simulink model "Model_Platform"  (R2018a)
settings: Solver=ode1  StartTime=0.0  StopTime=inf  FixedStep=0.001  RelTol=1e-3  EnableMultiTasking=on
PreLoadFcn:
  | ;HLABlocksetInit;;HLABlocksetInit;;HLABlocksetInit;
PostLoadFcn:
  | ;set_param(gcs,'PostCodeGenCommand', 'rtw_defines(buildInfo)');;set_param(gcs,'PostCodeGenCommand', 'rtw_defines(buildInfo)');;set_param(gcs,'PostCodeGenCommand', 'rtw_defines(buildInfo)');
undefined symbols (not defined in the file or in its folder): eng_speed, Heading_init, inertiaLateral, Joystick, Newton, omega_engine, omega_max, omega_wheel, Para, radiusWheel, Raphson, Standard_Devices, torque, Torque_lost, Torque_lost_wheel, X_init, Y_init, Z_init
libraries: simulink x26, dspnetwork x4, rtwinlib x2, PC_Simulator_Lib x2, vrlib x1
(part 2 of 4)

== system Model_Platform/Vehicle model/Vehicle dynamics/velocity ==
  longitudenal_velocity_Vx : Inport
  Lateral_velocity_Vy : Inport  Port=2
  rate_of_change_Yaw_Angle : Inport  Port=3
  angel_of_rotation_of_front_left_wheel : Inport  Port=4
  angel_of_rotation_of_front_Right_wheel : Inport  Port=5
  Mux2 : Mux
  Mux3 : Mux
  R : Subsystem
  to_tire : Subsystem
  velocity_at_Front_Left : Subsystem
  velocity_at_Front_Right : Subsystem
  velocity_at_Rear_Left : Subsystem
  velocity_at_Rear_Right : Subsystem
  velocity_conditioning : Subsystem
  velocity_at_wheels_in_X_mux(4) : Outport
  velocity_at_wheels_in_Y_mux(4) : Outport  Port=2
  R_CG : Outport  Port=3
  wires:
  velocity_conditioning/3(R_CGout) -> R_CG/1
  to_tire/2(velocity_at_wheels_in_Y_mux(4)final) -> velocity_at_wheels_in_Y_mux(4)/1
  to_tire/1(velocity_at_wheels_in_X_mux(4)final) -> velocity_at_wheels_in_X_mux(4)/1
  angel_of_rotation_of_front_Right_wheel/1 -> to_tire/2(angel_of_rotation_of_front_Right_wheel)
  angel_of_rotation_of_front_left_wheel/1 -> to_tire/1(angel_of_rotation_of_front_left_wheel)
  velocity_conditioning/1(velocity_at_wheels_in_X_mux(4)out) -> to_tire/3(velocity_at_wheels_in_X_mux(4))
  velocity_conditioning/2(velocity_at_wheels_in_Y_mux(4)out) -> to_tire/4(velocity_at_wheels_in_Y_mux(4))
  Mux2/1 -> velocity_conditioning/1(velocity_at_wheels_in_X_mux(4)in)
  Mux3/1 -> velocity_conditioning/2(velocity_at_wheels_in_Y_mux(4)in)
  R/1(R_CG) -> velocity_conditioning/3(R_CGin)
  Lateral_velocity_Vy/1 -> velocity_conditioning/5(VyCG), velocity_at_Front_Right/3(Lateral_velocity_Vy), R/3(Lateral_velocity_Vy), velocity_at_Rear_Right/3(Lateral_velocity_Vy), velocity_at_Rear_Left/3(Lateral_velocity_Vy), velocity_at_Front_Left/3(Lateral_velocity_Vy)
  velocity_at_Rear_Left/3(slip_angel_at_Rear_left) -> R/1(slip_angel_at_Rear_left)
  velocity_at_Rear_Right/2(velocity_at_Rear_Right_in_Y) -> Mux3/4
  velocity_at_Rear_Left/2(velocity_at_Rear_left_in_Y) -> Mux3/3
  velocity_at_Front_Left/2(velocity_at_Front_left_in_Y) -> Mux3/1
  velocity_at_Front_Right/2(velocity_at_Front_Right_in_Y) -> Mux3/2
  velocity_at_Rear_Right/1(velocity_at_Rear_Right_in_X) -> Mux2/4
  velocity_at_Rear_Left/1(velocity_at_Rear_left_in_X) -> Mux2/3
  velocity_at_Front_Right/1(velocity_at_Front_Right_in_X) -> Mux2/2
  velocity_at_Front_Left/1(velocity_at_Front_left_in_X) -> Mux2/1
  longitudenal_velocity_Vx/1 -> velocity_conditioning/4(VxCG), velocity_at_Front_Right/2(longitudenal_velocity_Vx), R/2(longitudenal_velocity_Vx), velocity_at_Rear_Right/2(longitudenal_velocity_Vx), velocity_at_Rear_Left/2(longitudenal_velocity_Vx), velocity_at_Front_Left/2(longitudenal_velocity_Vx)
  rate_of_change_Yaw_Angle/1 -> velocity_at_Front_Right/1(rate_of_change_Yaw_Angle), velocity_at_Rear_Right/1(rate_of_change_Yaw_Angle), velocity_at_Rear_Left/1(rate_of_change_Yaw_Angle), velocity_at_Front_Left/1(rate_of_change_Yaw_Angle)

== system Model_Platform/Vehicle model/Vehicle dynamics/xy_Global ==
  note: yaw_vehicle
  Vx_CG : Inport
  Vy_CG : Inport  Port=2
  rate_of_change_Yaw_Angle : Inport  Port=3
  Add8 : Sum  Inputs=+-
  Add9 : Sum
  Integrator1 : Integrator  InitialCondition=Heading_init
  Integrator8 : Integrator  InitialCondition=X_init
  Integrator9 : Integrator  InitialCondition=Y_init
  Product{16..19} (4 alike) : Product  RndMeth=Zero
  Trigonometric Function : Trigonometry  Operator=cos
  Trigonometric Function1 : Trigonometry
  Vx_global : Outport
  Vy_global : Outport  Port=2
  x_CG : Outport  Port=3
  y_CG : Outport  Port=4
  Actual_YAW : Outport  Port=5
  wires:
  Add9/1 -> Vy_global/1, Integrator9/1
  Integrator8/1 -> x_CG/1
  rate_of_change_Yaw_Angle/1 -> Integrator1/1
  Integrator1/1 -> Trigonometric Function1/1, Trigonometric Function/1, Actual_YAW/1
  Vx_CG/1 -> Product16/1, Product18/1
  Vy_CG/1 -> Product17/1, Product19/2
  Add8/1 -> Vx_global/1, Integrator8/1
  Product16/1 -> Add8/1
  Product17/1 -> Add8/2
  Product19/1 -> Add9/2
  Product18/1 -> Add9/1
  Integrator9/1 -> y_CG/1
  Trigonometric Function/1 -> Product19/1, Product16/2
  Trigonometric Function1/1 -> Product17/2, Product18/2

== system Model_Platform/Vehicle model/Drive_Train/4_Wheels_drive_train_and_Brake/Brake ==
  Feedback : Inport
  Add : Sum
  Bus Selector1 : BusSelector  OutputSignals=Vehicle_Dynamics.Vx_COG[m|s]
  Bus Selector6 : BusSelector  OutputSignals=Driver_Interface.Brake_Pedal_norm
  Compare To Constant : simulink/Logic and Bit Operations/Compare To Constant  relop=>=  const=0.7  OutDataTypeStr=uint8
  Compare To Constant1 : simulink/Logic and Bit Operations/Compare To Constant  relop=<=  const=-1  OutDataTypeStr=uint8
  Compare To Constant2 : simulink/Logic and Bit Operations/Compare To Constant  relop=<  const=0  OutDataTypeStr=uint8
  Constant1 : Constant  Value=0.35
  Constant2 : Constant
  Data Type Conversion : DataTypeConversion
  Data Type Conversion1 : DataTypeConversion
  Ground : Ground
  Ground1 : Ground
  Logical Operator : Logic  Operator=OR  AllPortsSameDT=off  OutDataTypeStr=boolean
  Product : Product  Inputs=5  RndMeth=Zero
  Product1 : Product  RndMeth=Zero
  Saturation : Saturate  UpperLimit=1  LowerLimit=0
  Sign : Signum
  Subsystem : Subsystem
  Subsystem1 : Subsystem
  Switch : Switch  Criteria=u2 > Threshold
  Terminator : Terminator
  Torque_max : Constant  Value=Para.DT.Torque_max_Brake.v
  Torque_Brake_Nm : Outport
  wires:
  Subsystem1/1(Out1) -> Add/2
  Add/1 -> Torque_Brake_Nm/1
  Product/1 -> Add/1
  Compare To Constant1/1 -> Logical Operator/2
  Data Type Conversion/1 -> Product/3
  Constant2/1 -> Switch/3, Product/5
  Switch/1 -> Product/4
  Product1/1 -> Product/1
  Constant1/1 -> Switch/1
  Data Type Conversion1/1 -> Switch/2
  Compare To Constant2/1 -> Data Type Conversion1/1
  Saturation/1 -> Subsystem1/2(Brake_Pedal[norm]), Product1/2
  Torque_max/1 -> Product1/1
  Feedback/1 -> Bus Selector6/1, Bus Selector1/1
  Bus Selector1/1 -> Sign/1, Compare To Constant2/1, Subsystem1/1(v_X_CoG[m|s]), Compare To Constant1/1, Compare To Constant/1  "<Vx_COG[m|s]>"
  Sign/1 -> Product/2
  Bus Selector6/1 -> Saturation/1  "<Brake_Pedal_norm>"
  Compare To Constant/1 -> Logical Operator/1
  Logical Operator/1 -> Data Type Conversion/1
  Subsystem/1(Torque_Brake_act_Nm) -> Terminator/1
  Ground/1 -> Subsystem/1(Torque_Brake_Nm)
  Ground1/1 -> Subsystem/2(Omega_rad/s)

== system Model_Platform/Vehicle model/Drive_Train/4_Wheels_drive_train_and_Brake/FL ==
  F_z : Inport
  Vx : Inport  Port=2
  Vy : Inport  Port=3
  Coeffecient_of_friction : Inport  Port=4
  Torque_Drive_Nm : Inport  Port=5
  Torque_Brake_Nm : Inport  Port=6
  Alpha_Kappa_Selector2 : Subsystem
  Fx_calculator : MATLAB Function  TreatAsAtomicUnit=on
  Fy_calculator : MATLAB Function  TreatAsAtomicUnit=on
  Radius_of_tire : Constant  Value=radiusWheel
  Wheel dynamics : Subsystem
  Fx : Outport
  Fy : Outport  Port=2
  Omega : Outport  Port=3
  omegaDot_radPs2 : Outport  Port=4
  wires:
  Alpha_Kappa_Selector2/2(alpha) -> Fx_calculator/2(alpha), Fy_calculator/2(alpha)
  Alpha_Kappa_Selector2/1(kappa) -> Fy_calculator/1(lambda), Fx_calculator/1(lambda)
  Torque_Brake_Nm/1 -> Wheel dynamics/3(Torque_Brake_Nm)
  Torque_Drive_Nm/1 -> Wheel dynamics/2(Torque_Drive_Nm)
  Wheel dynamics/2(omegaDot_radPs2) -> omegaDot_radPs2/1
  Fx_calculator/1(Fx) -> Alpha_Kappa_Selector2/5(Fx), Fx/1, Wheel dynamics/1(F_x)  "F_long"
  Coeffecient_of_friction/1 -> Fx_calculator/4(mue), Fy_calculator/5(mue)
  Fy_calculator/1(Fy) -> Fy/1
  F_z/1 -> Fx_calculator/3(Fz), Fy_calculator/4(Fz)
  Vy/1 -> Alpha_Kappa_Selector2/2(Vy)
  Radius_of_tire/1 -> Alpha_Kappa_Selector2/4(Rdyn)
  Vx/1 -> Alpha_Kappa_Selector2/1(Vx), Fy_calculator/3(V_x)
  Wheel dynamics/1(omega_radPs) -> Alpha_Kappa_Selector2/3(omega), Omega/1

== system Model_Platform/Vehicle model/Drive_Train/4_Wheels_drive_train_and_Brake/FR ==
  F_z : Inport
  Vx : Inport  Port=2
  Vy : Inport  Port=3
  Coeffecient_of_friction : Inport  Port=4
  Torque_Drive_Nm : Inport  Port=5
  Torque_Brake_Nm : Inport  Port=6
  Alpha_Kappa_Selector2 : Subsystem
  Fx_calculator : MATLAB Function  TreatAsAtomicUnit=on
  Fy_calculator : MATLAB Function  TreatAsAtomicUnit=on
  Radius_of_tire : Constant  Value=radiusWheel
  Wheel dynamics : Subsystem
  Fx : Outport
  Fy : Outport  Port=2
  Omega : Outport  Port=3
  omegaDot_radPs2 : Outport  Port=4
  wires:
  Torque_Brake_Nm/1 -> Wheel dynamics/3(Torque_Brake_Nm)
  Torque_Drive_Nm/1 -> Wheel dynamics/2(Torque_Drive_Nm)
  Wheel dynamics/2(omegaDot_radPs2) -> omegaDot_radPs2/1
  Fx_calculator/1(Fx) -> Fx/1, Wheel dynamics/1(F_x), Alpha_Kappa_Selector2/5(Fx)  "F_long"
  Coeffecient_of_friction/1 -> Fx_calculator/4(mue), Fy_calculator/5(mue)
  Fy_calculator/1(Fy) -> Fy/1
  Alpha_Kappa_Selector2/1(kappa) -> Fx_calculator/1(lambda), Fy_calculator/1(lambda)
  Alpha_Kappa_Selector2/2(alpha) -> Fy_calculator/2(alpha), Fx_calculator/2(alpha)
  F_z/1 -> Fx_calculator/3(Fz), Fy_calculator/4(Fz)
  Vy/1 -> Alpha_Kappa_Selector2/2(Vy)
  Radius_of_tire/1 -> Alpha_Kappa_Selector2/4(Rdyn)
  Vx/1 -> Fy_calculator/3(V_x), Alpha_Kappa_Selector2/1(Vx)
  Wheel dynamics/1(omega_radPs) -> Omega/1, Alpha_Kappa_Selector2/3(omega)

== system Model_Platform/Vehicle model/Drive_Train/4_Wheels_drive_train_and_Brake/RL ==
  F_z : Inport
  Vx : Inport  Port=2
  Vy : Inport  Port=3
  Coeffecient_of_friction : Inport  Port=4
  Torque_Drive_Nm : Inport  Port=5
  Torque_Brake_Nm : Inport  Port=6
  Alpha_Kappa_Selector2 : Subsystem
  Fx_calculator : MATLAB Function  TreatAsAtomicUnit=on
  Fy_calculator : MATLAB Function  TreatAsAtomicUnit=on
  Radius_of_tire : Constant  Value=radiusWheel
  Wheel dynamics : Subsystem
  Fx : Outport
  Fy : Outport  Port=2
  Omega : Outport  Port=3
  omegaDot_radPs2 : Outport  Port=4
  wires:
  Torque_Brake_Nm/1 -> Wheel dynamics/3(Torque_Brake_Nm)
  Torque_Drive_Nm/1 -> Wheel dynamics/2(Torque_Drive_Nm)
  Wheel dynamics/2(omegaDot_radPs2) -> omegaDot_radPs2/1
  Fx_calculator/1(Fx) -> Alpha_Kappa_Selector2/5(Fx), Fx/1, Wheel dynamics/1(F_x)  "F_long"
  Coeffecient_of_friction/1 -> Fx_calculator/4(mue), Fy_calculator/5(mue)
  Fy_calculator/1(Fy) -> Fy/1
  Alpha_Kappa_Selector2/1(kappa) -> Fx_calculator/1(lambda), Fy_calculator/1(lambda)
  Alpha_Kappa_Selector2/2(alpha) -> Fy_calculator/2(alpha), Fx_calculator/2(alpha)
  F_z/1 -> Fx_calculator/3(Fz), Fy_calculator/4(Fz)
  Vy/1 -> Alpha_Kappa_Selector2/2(Vy)
  Radius_of_tire/1 -> Alpha_Kappa_Selector2/4(Rdyn)
  Vx/1 -> Fy_calculator/3(V_x), Alpha_Kappa_Selector2/1(Vx)
  Wheel dynamics/1(omega_radPs) -> Alpha_Kappa_Selector2/3(omega), Omega/1

== system Model_Platform/Vehicle model/Drive_Train/4_Wheels_drive_train_and_Brake/RR ==
  F_z : Inport
  Vx : Inport  Port=2
  Vy : Inport  Port=3
  Coeffecient_of_friction : Inport  Port=4
  Torque_Drive_Nm : Inport  Port=5
  Torque_Brake_Nm : Inport  Port=6
  Alpha_Kappa_Selector2 : Subsystem
  Fx_calculator : MATLAB Function  TreatAsAtomicUnit=on
  Fy_calculator : MATLAB Function  TreatAsAtomicUnit=on
  Radius_of_tire : Constant  Value=radiusWheel
  Wheel dynamics : Subsystem
  Fx : Outport
  Fy : Outport  Port=2
  Omega : Outport  Port=3
  omegaDot_radPs2 : Outport  Port=4
  wires:
  Torque_Brake_Nm/1 -> Wheel dynamics/3(Torque_Brake_Nm)
  Torque_Drive_Nm/1 -> Wheel dynamics/2(Torque_Drive_Nm)
  Wheel dynamics/2(omegaDot_radPs2) -> omegaDot_radPs2/1
  Fx_calculator/1(Fx) -> Alpha_Kappa_Selector2/5(Fx), Fx/1, Wheel dynamics/1(F_x)  "F_long"
  Coeffecient_of_friction/1 -> Fx_calculator/4(mue), Fy_calculator/5(mue)
  Fy_calculator/1(Fy) -> Fy/1
  Alpha_Kappa_Selector2/1(kappa) -> Fx_calculator/1(lambda), Fy_calculator/1(lambda)
  Alpha_Kappa_Selector2/2(alpha) -> Fy_calculator/2(alpha), Fx_calculator/2(alpha)
  F_z/1 -> Fx_calculator/3(Fz), Fy_calculator/4(Fz)
  Vy/1 -> Alpha_Kappa_Selector2/2(Vy)
  Radius_of_tire/1 -> Alpha_Kappa_Selector2/4(Rdyn)
  Vx/1 -> Alpha_Kappa_Selector2/1(Vx), Fy_calculator/3(V_x)
  Wheel dynamics/1(omega_radPs) -> Alpha_Kappa_Selector2/3(omega), Omega/1

== system Model_Platform/Vehicle model/HMI_Realtime_normal_mode/HMI_Logitech1/Subsystem1 ==
  In1 : Inport
  Compare To Constant : simulink/Logic and Bit Operations/Compare To Constant  relop=>=  const=0.0001  OutDataTypeStr=boolean
  Constant : Constant
  Data Type Conversion : DataTypeConversion
  Gain : Gain
  Product : Product
  Sum : Sum  Inputs=|-+
  Out1 : Outport
  wires:
  Data Type Conversion/1 -> Product/2
  Compare To Constant/1 -> Data Type Conversion/1
  Product/1 -> Out1/1
  In1/1 -> Sum/1
  Sum/1 -> Gain/1
  Constant/1 -> Sum/2
  Gain/1 -> Product/1, Compare To Constant/1

== system Model_Platform/Vehicle model/HMI_Realtime_normal_mode/HMI_Logitech1/Subsystem2 ==
  In1 : Inport
  Compare To Constant : simulink/Logic and Bit Operations/Compare To Constant  relop=>=  const=0.0001  OutDataTypeStr=boolean
  Constant : Constant
  Data Type Conversion : DataTypeConversion
  Gain : Gain  Gain=.5
  Product : Product
  Sum : Sum  Inputs=|-+
  Out1 : Outport
  wires:
  Data Type Conversion/1 -> Product/2
  Compare To Constant/1 -> Data Type Conversion/1
  Product/1 -> Out1/1
  In1/1 -> Sum/1
  Sum/1 -> Gain/1
  Constant/1 -> Sum/2
  Gain/1 -> Product/1, Compare To Constant/1

== system Model_Platform/Vehicle model/Vehicle dynamics/Forces_transformation/Force_of_Aerodynamics ==
  note: Neglecting the air resistance effect in Y and modefing the equation
      | (V_abs*cos(slip))^2*Cd
      | insted of
      | V_abs^2*cos(slip)*Cd
      | by Berry
      | if not understud call me now
      | +20122299183
  velocity_of_car_absolut : Inport
  Slip_angle_of_velocity : Inport  Port=2
  Demux : Demux  Outputs=2
  Gain : Gain  Gain=Para.VD.Air_Risistance_Coefficient.v
  Product1 : Product  RndMeth=Zero
  Product2 : Product  RndMeth=Zero
  Product4 : Product  RndMeth=Zero
  Trigonometric Function3 : Trigonometry  Operator=cos
  Unary Minus : UnaryMinus
  Force_of_aerodynamics_in_X : Outport
  wires:
  Product2/1 -> Force_of_aerodynamics_in_X/1
  Gain/1 -> Product2/1
  Unary Minus/1 -> Product2/2
  Demux/2 -> Unary Minus/1
  Demux/1 -> Product4/1
  velocity_of_car_absolut/1 -> Demux/1
  Product1/1 -> Gain/1
  Product4/1 -> Product1/1, Product1/2
  Slip_angle_of_velocity/1 -> Trigonometric Function3/1
  Trigonometric Function3/1 -> Product4/2

== system Model_Platform/Vehicle model/Vehicle dynamics/Forces_transformation/Moment _about _Z_axis_calculation ==
  note: produce
      | the moment around Z
      | axis due to the total effect
      | of the forces acting on the
      | vehicle
  note: RR_Y
  note: RL_Y
  note: FR_Y
  note: FL_Y
  note: RR_X
  note: RL_X
  note: FR_X
  note: FL_X
  Forces_Acting_in_X_Wheels : Inport
  Forces_Acting_in_Y_Wheels : Inport  Port=2
  Add : Sum  Inputs=-++-
  Demux1 : Demux
  Demux3 : Demux
  Length_CG_Front_Wheels : Constant  Value=Para.VD.Length_Front.v
  Length_CG_Rear_Wheels : Constant  Value=Para.VD.Length_Rear.v
  Product{1..4} (4 alike) : Product  RndMeth=Zero
  Subtract{1..4} (4 alike) : Sum
  Width_of_Car/2 : Constant  Value=Para.VD.Wheel_Base_Width.v/2
  Moment _about _Z_axis : Outport
  wires:
  Add/1 -> Moment _about _Z_axis/1
  Demux3/2 -> Subtract3/1
  Demux3/3 -> Subtract4/2
  Length_CG_Rear_Wheels/1 -> Product2/2
  Length_CG_Front_Wheels/1 -> Product1/2
  Forces_Acting_in_Y_Wheels/1 -> Demux1/1
  Forces_Acting_in_X_Wheels/1 -> Demux3/1
  Width_of_Car/2/1 -> Product4/1, Product3/1
  Demux3/4 -> Subtract3/2
  Demux3/1 -> Subtract4/1
  Subtract4/1 -> Product3/2
  Subtract3/1 -> Product4/2
  Product4/1 -> Add/2
  Product3/1 -> Add/1
  Product2/1 -> Add/4
  Product1/1 -> Add/3
  Subtract1/1 -> Product2/1
  Demux1/4 -> Subtract1/2
  Demux1/3 -> Subtract1/1
  Subtract2/1 -> Product1/1
  Demux1/2 -> Subtract2/2
  Demux1/1 -> Subtract2/1

== system Model_Platform/Vehicle model/Vehicle dynamics/Forces_transformation/Moment _about _x_axis_calculation ==
  note: the total effect of forces
      | acting as a moment
      | around the X axis
  note: RR_Y
  note: RL_Y
  note: FR_Y
  note: FL_Y
  note: RR_Z
  note: RL_Z
  note: FR_Z
  note: FL_Z
  Forces_Z_Wheels : Inport
  Forces_Y_Wheels : Inport  Port=2
  Hight_Front_Left : Inport  Port=3
  Hight_Front_Right : Inport  Port=4
  Hight_Rear_Left : Inport  Port=5
  Hight_Rear_Right : Inport  Port=6
  Add1 : Sum  Inputs=+-+-
  Add2 : Sum  Inputs=++++
  Add3 : Sum
  Demux2 : Demux
  Demux3 : Demux
  Divide{9..16} (8 alike) : Product  Inputs=**
  Width_of_Car/1 : Constant  Value=Para.VD.Wheel_Base_Width.v/2
  Moment _about _X_axis1 : Outport
  wires:
  Add3/1 -> Moment _about _X_axis1/1
  Add2/1 -> Add3/2
  Add1/1 -> Add3/1
  Hight_Rear_Right/1 -> Divide16/2
  Hight_Rear_Left/1 -> Divide15/2
  Hight_Front_Right/1 -> Divide14/2
  Hight_Front_Left/1 -> Divide13/2
  Forces_Y_Wheels/1 -> Demux3/1
  Demux3/4 -> Divide16/1
  Demux3/3 -> Divide15/1
  Demux3/2 -> Divide14/1
  Demux3/1 -> Divide13/1
  Divide16/1 -> Add2/4
  Divide15/1 -> Add2/3
  Divide14/1 -> Add2/2
  Divide13/1 -> Add2/1
  Forces_Z_Wheels/1 -> Demux2/1
  Demux2/4 -> Divide12/2
  Demux2/3 -> Divide11/2
  Demux2/2 -> Divide10/2
  Demux2/1 -> Divide9/2
  Width_of_Car/1/1 -> Divide12/1, Divide11/1, Divide10/1, Divide9/1
  Divide9/1 -> Add1/1
  Divide10/1 -> Add1/2
  Divide11/1 -> Add1/3
  Divide12/1 -> Add1/4

== system Model_Platform/Vehicle model/Vehicle dynamics/Forces_transformation/Moment _about _y_axis_calculation ==
  note: the total effect of the car forces
      | represented as a moment acting on the
      | CG around Y axis
  note: RR_X
  note: RL_X
  note: FR_X
  note: FL_X
  note: RR_Z
  note: RL_Z
  note: FR_Z
  note: FL_Z
  Forces_Z_Wheels : Inport
  Forces_X_Wheels : Inport  Port=2
  Hight_Front_Left : Inport  Port=3
  Hight_Front_Right : Inport  Port=4
  Hight_Rear_Left : Inport  Port=5
  Hight_Rear_Right : Inport  Port=6
  Add1 : Sum  Inputs=--++
  Add2 : Sum  Inputs=----
  Add3 : Sum
  Demux1 : Demux
  Demux9 : Demux
  Divide{8..15} (8 alike) : Product  Inputs=**
  Length_CG_Front_Wheels : Constant  Value=Para.VD.Length_Front.v
  Length_CG_Rear_Wheels : Constant  Value=Para.VD.Length_Rear.v
  Moment _about _Y_axis2 : Outport
  wires:
  Add3/1 -> Moment _about _Y_axis2/1
  Hight_Rear_Right/1 -> Divide15/2
  Hight_Rear_Left/1 -> Divide14/2
  Hight_Front_Right/1 -> Divide13/2
  Hight_Front_Left/1 -> Divide12/2
  Forces_X_Wheels/1 -> Demux1/1
  Demux1/4 -> Divide15/1
  Demux1/3 -> Divide14/1
  Demux1/2 -> Divide13/1
  Demux1/1 -> Divide12/1
  Forces_Z_Wheels/1 -> Demux9/1
  Length_CG_Rear_Wheels/1 -> Divide11/2, Divide10/2
  Length_CG_Front_Wheels/1 -> Divide9/2, Divide8/2
  Demux9/4 -> Divide11/1
  Demux9/3 -> Divide10/1
  Demux9/2 -> Divide9/1
  Demux9/1 -> Divide8/1
  Divide15/1 -> Add2/4
  Divide14/1 -> Add2/3
  Divide13/1 -> Add2/2
  Divide12/1 -> Add2/1
  Divide11/1 -> Add1/4
  Divide10/1 -> Add1/3
  Divide9/1 -> Add1/2
  Divide8/1 -> Add1/1
  Add2/1 -> Add3/2
  Add1/1 -> Add3/1

== system Model_Platform/Vehicle model/Vehicle dynamics/Forces_transformation/Z1-->angles ==
  Z1(4) : Inport
  Constant3 : Constant  Value=-2*Para.VD.Length_Front.v
  Constant4 : Constant  Value=Para.VD.Wheel_Base_Width.v
  Demux : Demux
  Divide : Product  Inputs=*/
  Divide1 : Product  Inputs=*/
  Subtract3 : Sum  Inputs=+-
  Subtract4 : Sum  Inputs=+-
  Terminator : Terminator
  Trigonometric Function1 : Trigonometry  Operator=asin
  Trigonometric Function2 : Trigonometry  Operator=asin
  Roll_angel(z1)1 : Outport
  Pitch_angel(z1) : Outport  Port=2
  wires:
  Demux/4 -> Terminator/1
  Z1(4)/1 -> Demux/1
  Demux/1 -> Subtract3/1, Subtract4/1
  Demux/3 -> Subtract3/2
  Subtract3/1 -> Divide/1
  Constant3/1 -> Divide/2
  Divide/1 -> Trigonometric Function1/1
  Trigonometric Function1/1 -> Pitch_angel(z1)/1
  Demux/2 -> Subtract4/2
  Subtract4/1 -> Divide1/1
  Constant4/1 -> Divide1/2
  Divide1/1 -> Trigonometric Function2/1
  Trigonometric Function2/1 -> Roll_angel(z1)1/1

== system Model_Platform/Vehicle model/Vehicle dynamics/Forces_transformation/force acting in X direction ==
  note: the summation of forces
      | acting on the X direction
      | on CG
  note: Force_rear_right_in_x
  note: Force_rear_left_in_x
  note: Force_Front_Right_in_x
  note: Force_Front_Left_in_x
  Forces_Acting_In_X_Wheel : Inport
  Force_acting_in_x_from_mass : Inport  Port=2
  Force_in_x_air : Inport  Port=3
  Add : Sum  Inputs=++++++
  Demux1 : Demux
  Force_acting_on_CG_in_x : Outport
  wires:
  Add/1 -> Force_acting_on_CG_in_x/1
  Forces_Acting_In_X_Wheel/1 -> Demux1/1
  Force_in_x_air/1 -> Add/6
  Force_acting_in_x_from_mass/1 -> Add/5
  Demux1/4 -> Add/4
  Demux1/3 -> Add/3
  Demux1/2 -> Add/2
  Demux1/1 -> Add/1

== system Model_Platform/Vehicle model/Vehicle dynamics/Forces_transformation/force acting in Y direction ==
  note: the summation of forces
      | acting on the Y direction
      | on CG
  note: Force_Rear_Right_in_Y
  note: Force_Rear_Left_in_Y
  note: Force_Front_Right_in_Y
  note: Force_Front_Left_in_Y
  Forces_Acting_In_Y_Wheels : Inport
  Force_From_Mass_Y : Inport  Port=2
  Add : Sum  Inputs=+++++
  Demux2 : Demux
  Force_acting_on_CG_in_Y : Outport
  wires:
  Add/1 -> Force_acting_on_CG_in_Y/1
  Forces_Acting_In_Y_Wheels/1 -> Demux2/1
  Demux2/1 -> Add/1
  Demux2/2 -> Add/2
  Demux2/3 -> Add/3
  Demux2/4 -> Add/4
  Force_From_Mass_Y/1 -> Add/5

== system Model_Platform/Vehicle model/Vehicle dynamics/Forces_transformation/force acting in Z direction ==
  note: the summation of forces acting
      | on CG in Z direction
  Forces_Z_Wheel : Inport
  Force_Mass_Z : Inport  Port=2
  Add : Sum  Inputs=+++++
  Demux5 : Demux
  Force_acting_on_CG_in_z : Outport
  wires:
  Forces_Z_Wheel/1 -> Demux5/1
  Force_Mass_Z/1 -> Add/5
  Demux5/4 -> Add/4
  Add/1 -> Force_acting_on_CG_in_z/1
  Demux5/3 -> Add/3
  Demux5/2 -> Add/2
  Demux5/1 -> Add/1

== system Model_Platform/Vehicle model/Vehicle dynamics/Forces_transformation/inclination_effect_on_mass ==
  note: FZ_due to roll
  Roll_angle(z1) : Inport
  Pitch_angel(z1) : Inport  Port=2
  Gain : Gain  Gain=-1
  Gain1 : Gain  Gain=-1
  Product{1..4} (4 alike) : Product  RndMeth=Zero
  Trigonometric Function : Trigonometry  Operator=cos
  Trigonometric Function1 : Trigonometry  Operator=cos
  Trigonometric Function2 : Trigonometry
  Trigonometric Function3 : Trigonometry
  m * g : Constant  Value=Para.VD.Mass.v * Para.VD.gravity.v
  FZ_due_to_mass : Outport
  Fx_due_to_mass : Outport  Port=2
  Fy_due_to_mass : Outport  Port=3
  wires:
  Product1/1 -> Product4/2
  Trigonometric Function/1 -> Product4/1
  Gain1/1 -> Product1/2
  Trigonometric Function1/1 -> Gain1/1
  Product2/1 -> Fx_due_to_mass/1
  Product4/1 -> FZ_due_to_mass/1
  Gain/1 -> Fy_due_to_mass/1
  Product3/1 -> Gain/1
  Trigonometric Function3/1 -> Product3/2
  Trigonometric Function2/1 -> Product2/1
  m * g/1 -> Product2/2, Product3/1, Product1/1
  Roll_angle(z1)/1 -> Trigonometric Function3/1, Trigonometric Function1/1
  Pitch_angel(z1)/1 -> Trigonometric Function2/1, Trigonometric Function/1

== system Model_Platform/Vehicle model/Vehicle dynamics/Horizontal_Dyn/Beta_Slip_Angle_calculation ==
  note: this block is to develop the beta
      | slip angle and the absolut speed
      | with which the vehicle travels
      | considering direction of traveling
  Longitudinal_Velocity_Vx : Inport
  Longitudinal_Velocity_Vy : Inport  Port=2
  Bus Creator : BusCreator  Inputs=2
  Divide1 : Product  Inputs=/*
  Divide2 : Product  Inputs=**
  Divide3 : Product  Inputs=**
  Math Function : Math  Operator=sqrt  SaturateOnIntegerOverflow=on
  Sign : Signum
  Sum : Sum
  Trigonometric Function1 : Trigonometry  Operator=atan
  Beta_Slip_Angle : Outport
  absolute_velocity_of_car_with_direction : Outport  Port=2
  wires:
  Math Function/1 -> Bus Creator/1
  Bus Creator/1 -> absolute_velocity_of_car_with_direction/1
  Sign/1 -> Bus Creator/2
  Sum/1 -> Math Function/1
  Divide3/1 -> Sum/2
  Divide2/1 -> Sum/1
  Longitudinal_Velocity_Vy/1 -> Divide1/2, Divide3/2, Divide3/1
  Trigonometric Function1/1 -> Beta_Slip_Angle/1
  Divide1/1 -> Trigonometric Function1/1
  Longitudinal_Velocity_Vx/1 -> Divide2/1, Sign/1, Divide2/2, Divide1/1

== system Model_Platform/Vehicle model/Vehicle dynamics/Horizontal_Dyn/about_z_axis ==
  note: Yawddot
  Moment _about _Z_axis : Inport
  reset : Inport  Port=2
  1/Inertia_Vertical axis : Gain  Gain=1/Para.VD.Inertia_zz.v  OutDataTypeStr=double
  Integrator1 : Integrator  InitialCondition=Heading_init
  Integrator4 : Integrator  ExternalReset=level
  Yaw_Angular_ACC : Outport
  Yaw_angle_Velcity : Outport  Port=2
  Yaw_angle_(rad) : Outport  Port=3
  wires:
  reset/1 -> Integrator4/2
  Integrator4/1 -> Yaw_angle_Velcity/1, Integrator1/1
  Integrator1/1 -> Yaw_angle_(rad)/1
  1/Inertia_Vertical axis/1 -> Integrator4/1, Yaw_Angular_ACC/1
  Moment _about _Z_axis/1 -> 1/Inertia_Vertical axis/1

== system Model_Platform/Vehicle model/Vehicle dynamics/Horizontal_Dyn/in_x_direction ==
  note: XDDot
  Force_acting_on_CG_in_x : Inport
  Constant : Constant  Value=eps
  Integrator2 : Integrator  InitialCondition=eps
  Integrator3 : Integrator
  Mass : Gain  Gain=1/Para.VD.Mass.v
  Sum : Sum  Inputs=|++
  Longitudinal_Velocity_Vx : Outport
  Displacement_x : Outport  Port=2
  Acceleration_Ax : Outport  Port=3
  wires:
  Constant/1 -> Sum/2
  Sum/1 -> Mass/1
  Force_acting_on_CG_in_x/1 -> Sum/1
  Integrator2/1 -> Longitudinal_Velocity_Vx/1, Integrator3/1
  Mass/1 -> Acceleration_Ax/1, Integrator2/1
  Integrator3/1 -> Displacement_x/1

== system Model_Platform/Vehicle model/Vehicle dynamics/Horizontal_Dyn/in_y_direction ==
  note: YDDot
  note: Y
  note: YDot
  Force_acting_on_CG_in_y : Inport
  reset : Inport  Port=2
  Integrator2 : Integrator  ExternalReset=level
  Integrator3 : Integrator
  Mass : Gain  Gain=1/Para.VD.Mass.v
  Lateral_Velocity_Vy : Outport
  Displacement_y : Outport  Port=2
  Acceleration_Ay : Outport  Port=3
  wires:
  reset/1 -> Integrator2/2
  Integrator2/1 -> Lateral_Velocity_Vy/1, Integrator3/1
  Mass/1 -> Acceleration_Ay/1, Integrator2/1
  Force_acting_on_CG_in_y/1 -> Mass/1
  Integrator3/1 -> Displacement_y/1

== system Model_Platform/Vehicle model/Vehicle dynamics/Horizontal_Dyn/reset ==
  In1 : Inport
  Abs : Abs
  Compare To Constant : simulink/Logic and Bit Operations/Compare To Constant  relop=<=  const=0.5  OutDataTypeStr=boolean
  Out1 : Outport
  wires:
  Compare To Constant/1 -> Out1/1
  Abs/1 -> Compare To Constant/1
  In1/1 -> Abs/1

== system Model_Platform/Vehicle model/Vehicle dynamics/Horizontal_Dyn/reset1 ==
  In1 : Inport
  Abs : Abs
  Compare To Constant : simulink/Logic and Bit Operations/Compare To Constant  relop=<=  const=0.5  OutDataTypeStr=boolean
  Out1 : Outport
  wires:
  In1/1 -> Abs/1
  Abs/1 -> Compare To Constant/1
  Compare To Constant/1 -> Out1/1

== system Model_Platform/Vehicle model/Vehicle dynamics/Output_Maping/Subsystem1 ==
  Force_Suspention : Inport
  Bus Creator : BusCreator  Inputs=4
  Demux : Demux
  Fz_Wheel[N] : Outport
  wires:
  Bus Creator/1 -> Fz_Wheel[N]/1
  Demux/4 -> Bus Creator/4  "Fz_Wheel_RR[N]"
  Demux/3 -> Bus Creator/3  "Fz_Wheel_RL[N]"
  Demux/2 -> Bus Creator/2  "Fz_Wheel_FR[N]"
  Demux/1 -> Bus Creator/1  "Fz_Wheel_FL[N]"
  Force_Suspention/1 -> Demux/1

== system Model_Platform/Vehicle model/Vehicle dynamics/Output_Maping/Velocity_Wheels_Maping_Block ==
  Velocity_Wheels_X[m|s] : Inport
  Velocity_Wheels_Y[m|s] : Inport  Port=2
  Bus Creator : BusCreator  Inputs=4
  Bus Creator{3..5,7} (4 alike) : BusCreator  Inputs=2
  Demux1 : Demux
  Demux2 : Demux
  Velocity_Wheels[m|s] : Outport
  wires:
  Bus Creator/1 -> Velocity_Wheels[m|s]/1  "Velocity_Wheels[m|s]"
  Velocity_Wheels_Y[m|s]/1 -> Demux2/1
  Velocity_Wheels_X[m|s]/1 -> Demux1/1
  Demux2/4 -> Bus Creator7/2  "vy_RR"
  Demux1/4 -> Bus Creator7/1  "vx_RR[m|s]"
  Demux2/3 -> Bus Creator5/2  "vy_RL[m|s]"
  Demux1/3 -> Bus Creator5/1  "vx_RL[m|s]"
  Demux2/2 -> Bus Creator4/2  "vy_FR[m|s]"
  Demux1/2 -> Bus Creator4/1  "vx_FR[m|s]"
  Demux2/1 -> Bus Creator3/2  "vy_FL[m|s]"
  Demux1/1 -> Bus Creator3/1  "vx_FL[m|s]"
  Bus Creator7/1 -> Bus Creator/4  "v_RR[m|s]"
  Bus Creator5/1 -> Bus Creator/3  "v_RL[m|s]"
  Bus Creator4/1 -> Bus Creator/2  "v_FR[m|s]"
  Bus Creator3/1 -> Bus Creator/1  "v_FL[m|s]"

== system Model_Platform/Vehicle model/Vehicle dynamics/Vertical_Dyn./Invers_Trangnometric_conv ==
  Vertical_Displacement_Z_vehicle_corners_actual(4) : Inport
  Add3 : Sum  Inputs=++++-
  Constant3 : Constant  Value=-2*Para.VD.Length_Front.v
  Constant4 : Constant  Value=Para.VD.Wheel_Base_Width.v
  Constant5 : Constant  Value=2*Para.VD.Length_Rear.v-2*Para.VD.Length_Front.v
  Demux : Demux
  Divide : Product  Inputs=*/
  Divide1 : Product  Inputs=*/
  Gain1 : Gain  Gain=0.25
  Product3 : Product  RndMeth=Zero
  Subtract3 : Sum  Inputs=+-
  Subtract4 : Sum  Inputs=+-
  Trigonometric Function1 : Trigonometry  Operator=asin
  Trigonometric Function2 : Trigonometry  Operator=asin
  Vertical_Displacement_Z_CG_actual : Outport
  Roll_actual : Outport  Port=2
  Pitch_actual : Outport  Port=3
  wires:
  Gain1/1 -> Vertical_Displacement_Z_CG_actual/1
  Add3/1 -> Gain1/1
  Product3/1 -> Add3/5
  Constant5/1 -> Product3/2
  Demux/4 -> Add3/4
  Trigonometric Function2/1 -> Roll_actual/1
  Divide1/1 -> Trigonometric Function2/1
  Constant4/1 -> Divide1/2
  Subtract4/1 -> Divide1/1
  Demux/2 -> Add3/2, Subtract4/2
  Trigonometric Function1/1 -> Pitch_actual/1
  Divide/1 -> Product3/1, Trigonometric Function1/1
  Constant3/1 -> Divide/2
  Subtract3/1 -> Divide/1
  Demux/3 -> Add3/3, Subtract3/2
  Demux/1 -> Add3/1, Subtract4/1, Subtract3/1
  Vertical_Displacement_Z_vehicle_corners_actual(4)/1 -> Demux/1

== system Model_Platform/Vehicle model/Vehicle dynamics/Vertical_Dyn./Mass_Distribution ==
  note: Force acting on front wheels = (m*g*Rear_Length)/(Front_Length+Rear_Length)
      | Force acting on Rear wheels = m*g -  (m*g*Rear_Length)/(Front_Length+Rear_Length)
      | the mass are just dividing by the gravity
  note: RR_Z
  note: RL_Z
  note: FR_Z
  note: FL_Z
  note: Reaction_Force_Rear_Wheels
  note: Reaction_Force_Front_Wheels
  Mass*gravity_in_Z : Inport
  Abs : Abs
  Divide : Product  Inputs=*/
  Divide1 : Product  Inputs=*/
  Divide2 : Product  Inputs=*/
  Gain : Gain  Gain=0.5
  Gain1 : Gain  Gain=0.5
  Length_CG_Rear_Wheels : Constant  Value=Para.VD.Length_Rear.v
  Mass*gravity1 : Constant  Value=Para.VD.gravity.v*Para.VD.Mass.v
  Mux : Mux
  Mux1 : Mux
  Product : Product  RndMeth=Zero
  Subtract : Sum  Inputs=+-
  Terminator : Terminator
  Terminator1 : Terminator
  Wheel_Base_Length : Constant  Value=Para.VD.Wheel_Base_Length.v
  gravity : Constant  Value=Para.VD.gravity.v
  Forces_Z_Mass : Outport
  wires:
  Abs/1 -> Subtract/1, Product/1
  Mux1/1 -> Terminator/1
  Mass*gravity1/1 -> Terminator1/1
  gravity/1 -> Divide2/2, Divide1/2
  Divide1/1 -> Mux1/2, Mux1/1
  Divide2/1 -> Mux1/3, Mux1/4
  Mux/1 -> Forces_Z_Mass/1
  Gain1/1 -> Divide2/1, Mux/4, Mux/3
  Gain/1 -> Divide1/1, Mux/2, Mux/1
  Subtract/1 -> Gain1/1
  Divide/1 -> Gain/1, Subtract/2
  Wheel_Base_Length/1 -> Divide/2
  Product/1 -> Divide/1
  Length_CG_Rear_Wheels/1 -> Product/2
  Mass*gravity_in_Z/1 -> Abs/1

== system Model_Platform/Vehicle model/Vehicle dynamics/Vertical_Dyn./Trangnometric_conv ==
  note: RR
  note: RL
  note: FR
  note: FL
  note: 0.5*Lt*sin(Roll)
  note: Lr*sin(Pitch)
  note: Lf*sin(pitch)
  Vertical_Displacement_Z_CG : Inport
  Pitch : Inport  Port=2
  Roll : Inport  Port=3
  Add : Sum
  Add1 : Sum
  Add2 : Sum
  Constant : Constant  Value=Para.VD.Wheel_Base_Width.v
  Constant1 : Constant  Value=Para.VD.Length_Rear.v
  Constant2 : Constant  Value=Para.VD.Length_Front.v
  Gain : Gain  Gain=0.5
  Mux : Mux
  Product : Product  RndMeth=Zero
  Product1 : Product  RndMeth=Zero
  Product2 : Product  RndMeth=Zero
  Subtract : Sum  Inputs=+-
  Subtract1 : Sum  Inputs=+-
  Subtract2 : Sum  Inputs=+-
  Trigonometric Function : Trigonometry
  Trigonometric Function1 : Trigonometry
  Vertical_Displacement_Z_vehicle_corners(4) : Outport
  wires:
  Subtract2/1 -> Mux/4
  Add2/1 -> Mux/3
  Add1/1 -> Subtract2/1, Add2/2
  Subtract1/1 -> Mux/2
  Add/1 -> Mux/1
  Subtract/1 -> Subtract1/1, Add/2
  Vertical_Displacement_Z_CG/1 -> Add1/1, Subtract/1
  Product/1 -> Subtract2/2, Add2/1, Subtract1/2, Add/1
  Product2/1 -> Add1/2
  Product1/1 -> Subtract/2
  Constant2/1 -> Product1/1
  Constant1/1 -> Product2/1
  Trigonometric Function/1 -> Product1/2, Product2/2
  Trigonometric Function1/1 -> Product/1
  Gain/1 -> Product/2
  Roll/1 -> Trigonometric Function1/1
  Pitch/1 -> Trigonometric Function/1
  Constant/1 -> Gain/1
  Mux/1 -> Vertical_Displacement_Z_vehicle_corners(4)/1

== system Model_Platform/Vehicle model/Vehicle dynamics/Vertical_Dyn./Vertical_movement ==
  Vertical_Force_CG : Inport
  Moment_Y-axis_CG : Inport  Port=2
  Moment_X-axis_CG : Inport  Port=3
  1/Ixx : Gain  Gain=1/Para.VD.Inertia_xx.v
  1/Iyy : Gain  Gain=1/Para.VD.Inertia_yy.v
  1/mass : Gain  Gain=1/Para.VD.Mass.v
  Integrator{1..6} (6 alike) : Integrator
  Vertical_Displacement_Z_CG : Outport
  Pitch : Outport  Port=2
  Roll : Outport  Port=3
  Vertical_Velocity_Z_CG[m|s] : Outport  Port=4
  wires:
  Integrator1/1 -> Vertical_Displacement_Z_CG/1
  1/Ixx/1 -> Integrator5/1
  1/Iyy/1 -> Integrator3/1
  Integrator5/1 -> Integrator4/1
  Integrator3/1 -> Integrator2/1
  Integrator2/1 -> Pitch/1
  Integrator4/1 -> Roll/1
  Integrator6/1 -> Vertical_Velocity_Z_CG[m|s]/1, Integrator1/1
  1/mass/1 -> Integrator6/1
  Moment_X-axis_CG/1 -> 1/Ixx/1
  Moment_Y-axis_CG/1 -> 1/Iyy/1
  Vertical_Force_CG/1 -> 1/mass/1

== system Model_Platform/Vehicle model/Vehicle dynamics/Vertical_Dyn./suspention_System ==
  Vertical_Displacement_Z2_vehicle_corners(4) : Inport
  Vertical_Displacement_Z0(4) : Inport  Port=2
  intial_force_from_mass_Wheels(4) : Inport  Port=3
  Demux : Demux
  Demux1 : Demux
  Demux3 : Demux
  Mux{,1..3} (4 alike) : Mux
  Rear_Right_Suspention : Subsystem
  Rear_left_Suspention : Subsystem
  front_left_Suspention : Subsystem
  front_right_Suspention : Subsystem
  Force_Suspention(4) : Outport
  Hight_Suspention(4) : Outport  Port=2
  Z1(4) : Outport  Port=3
  Vertical_Displacement_Z_vehicle_corners_actual(4) : Outport  Port=4
  wires:
  Rear_Right_Suspention/4(Z2actual) -> Mux3/4
  Rear_left_Suspention/4(Z2actual) -> Mux3/3
  front_right_Suspention/4(Z2actual) -> Mux3/2
  front_left_Suspention/4(Z2actual) -> Mux3/1
  Mux3/1 -> Vertical_Displacement_Z_vehicle_corners_actual(4)/1
  Mux2/1 -> Z1(4)/1
  Rear_Right_Suspention/3(Z1) -> Mux2/4
  Rear_left_Suspention/3(Z1) -> Mux2/3
  front_right_Suspention/3(Z1) -> Mux2/2
  front_left_Suspention/3(Z1) -> Mux2/1
  front_right_Suspention/2(Hight_front_right) -> front_left_Suspention/4(Hight_front_right), Mux1/2
  front_left_Suspention/2(Hight_front_left) -> front_right_Suspention/4(Hight_front_left), Mux1/1
  front_right_Suspention/1(Force_Suspention_FR) -> Mux/2
  front_left_Suspention/1(Force_Suspention_FL) -> Mux/1
  Demux3/3 -> Rear_left_Suspention/3(intial_force_form_mass_rl)
  Demux3/2 -> front_right_Suspention/3(intial_force_form_mass_fr)
  Demux3/1 -> front_left_Suspention/3(intial_force_form_mass_fl)
  Demux1/3 -> Rear_left_Suspention/2(Vertical_Displacement_Z0)
  Demux1/2 -> front_right_Suspention/2(Vertical_Displacement_Z0)
  Demux1/1 -> front_left_Suspention/2(Vertical_Displacement_Z0)
  Demux/3 -> Rear_left_Suspention/1(Vertical_Displacement_Z_vehicle_corner_Rl)
  Demux/2 -> front_right_Suspention/1(Vertical_Displacement_Z_vehicle_corner_fr)
  Demux/1 -> front_left_Suspention/1(Vertical_Displacement_Z_vehicle_corner_fl)
  Rear_left_Suspention/1(Force_Suspention_RL) -> Mux/3
  Mux/1 -> Force_Suspention(4)/1
  Vertical_Displacement_Z2_vehicle_corners(4)/1 -> Demux/1
  Vertical_Displacement_Z0(4)/1 -> Demux1/1
  Mux1/1 -> Hight_Suspention(4)/1
  intial_force_from_mass_Wheels(4)/1 -> Demux3/1
  Rear_left_Suspention/2(Hight_Reer_left) -> Mux1/3
  Demux/4 -> Rear_Right_Suspention/1(Vertical_Displacement_Z_vehicle_corner_RR)
  Demux1/4 -> Rear_Right_Suspention/2(Vertical_Displacement_Z0)
  Demux3/4 -> Rear_Right_Suspention/3(intial_force_form_mass_rr)
  Rear_Right_Suspention/1(Force_Suspention_RR) -> Mux/4
  Rear_Right_Suspention/2(Hight_Reer_Right) -> Mux1/4

== system Model_Platform/Vehicle model/Vehicle dynamics/force_from_wheel_cordination_transformation/Steer_model ==
  note: this block is to analyze the
      | forces acting on the wheels
      |  coordination to find thier
      | components on the car coordination
      | -with respect to CAR XY-
  note: this block is to find the angle of rotation of
      | the front left and rear wheels
  note: To transform the front wheels forces to be calculated in the horizontal block
  note: FRxsin+FRycos
  note: FRxcos+FRysin
  note: FLxsin+FLycos
  note: FLxcos+FLysin
  Steering_Angle_HMI_[-1 1] : Inport
  FLx_T : Inport  Port=2
  FRx_T : Inport  Port=3
  FLy_T : Inport  Port=4
  FRy_T : Inport  Port=5
  Force_Analysis : Subsystem
  Steer_Angel_Distribution1 : Subsystem
  FLx : Outport
  FRx : Outport  Port=2
  FLy : Outport  Port=3
  FRy : Outport  Port=4
  FL_Angle : Outport  Port=5
  FR_Angle : Outport  Port=6
  wires:
  Steer_Angel_Distribution1/2(FR_Angle) -> Force_Analysis/2(FR_Angle), FR_Angle/1
  Steer_Angel_Distribution1/1(FL_Angle) -> Force_Analysis/1(FL_Angle), FL_Angle/1
  FRy_T/1 -> Force_Analysis/6(FRy_T)
  FLy_T/1 -> Force_Analysis/5(FLy_T)
  FRx_T/1 -> Force_Analysis/4(FRx_T)
  FLx_T/1 -> Force_Analysis/3(FLx_T)
  Force_Analysis/4(FRy) -> FRy/1
  Force_Analysis/3(FRx) -> FRx/1
  Force_Analysis/2(FLy) -> FLy/1
  Force_Analysis/1(FLx) -> FLx/1
  Steering_Angle_HMI_[-1 1]/1 -> Steer_Angel_Distribution1/1(Steering_Angle_HMI_[-1 1])

== system Model_Platform/Vehicle model/Vehicle dynamics/velocity/R ==
  note: just for test
  note: tan(betaCG)
  slip_angel_at_Rear_left : Inport
  longitudenal_velocity_Vx : Inport  Port=2
  Lateral_velocity_Vy : Inport  Port=3
  Divide2 : Product  Inputs=/*
  Length_CG_Rear_Wheels : Constant  Value=Para.VD.Length_Rear.v
  Product2 : Product  RndMeth=Zero
  Product3 : Product  RndMeth=Zero
  Product4 : Product  RndMeth=Zero
  Rcg : Math  Operator=sqrt  SaturateOnIntegerOverflow=on
  Subtract : Sum  Inputs=+-
  Subtract1 : Sum  Inputs=+-
  Sum3 : Sum  Inputs=|++
  Width_of_Car/2 : Constant  Value=Para.VD.Wheel_Base_Width.v/2
  la : Product  Inputs=*/
  ln : Product  RndMeth=Zero
  tanbetaRL : Trigonometry  Operator=tan
  R_CG : Outport
  wires:
  Rcg/1 -> R_CG/1
  Sum3/1 -> Rcg/1
  Product4/1 -> Sum3/2
  Product3/1 -> Sum3/1
  ln/1 -> Product3/2, Product3/1
  la/1 -> Product4/2, Product4/1, ln/1
  Subtract1/1 -> la/2
  Subtract/1 -> la/1
  Product2/1 -> Subtract/2
  Length_CG_Rear_Wheels/1 -> Subtract/1
  tanbetaRL/1 -> Subtract1/2, Product2/2
  Width_of_Car/2/1 -> Product2/1
  slip_angel_at_Rear_left/1 -> tanbetaRL/1
  Divide2/1 -> ln/2, Subtract1/1
  Lateral_velocity_Vy/1 -> Divide2/2
  longitudenal_velocity_Vx/1 -> Divide2/1

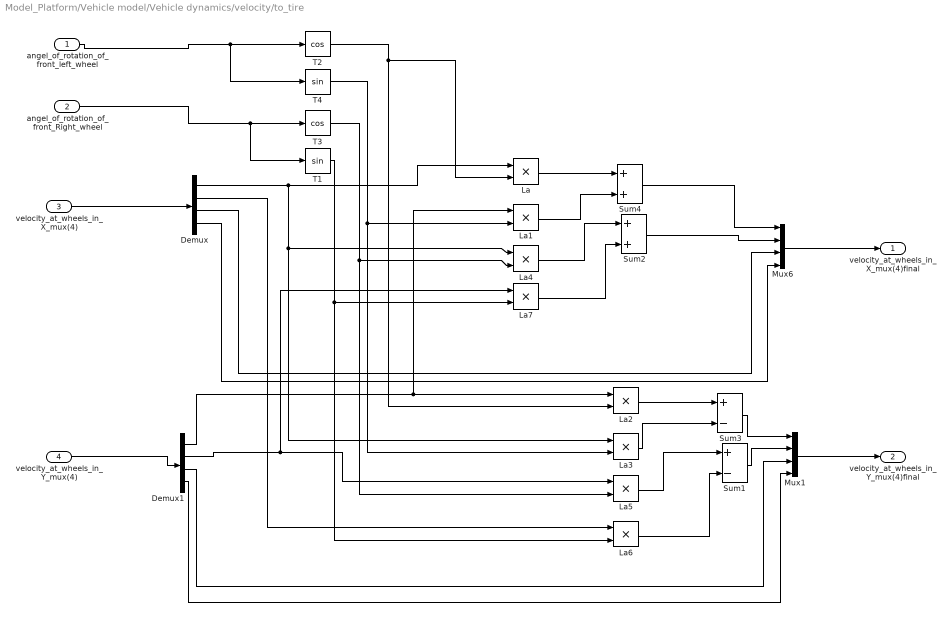
== system Model_Platform/Vehicle model/Vehicle dynamics/velocity/to_tire ==
  angel_of_rotation_of_front_left_wheel : Inport
  angel_of_rotation_of_front_Right_wheel : Inport  Port=2
  velocity_at_wheels_in_X_mux(4) : Inport  Port=3
  velocity_at_wheels_in_Y_mux(4) : Inport  Port=4
  Demux : Demux
  Demux1 : Demux
  La{,1..7} (8 alike) : Product  RndMeth=Zero
  Mux1 : Mux
  Mux6 : Mux
  Sum1 : Sum  Inputs=+-
  Sum2 : Sum
  Sum3 : Sum  Inputs=+-
  Sum4 : Sum
  T1 : Trigonometry
  T2 : Trigonometry  Operator=cos
  T3 : Trigonometry  Operator=cos
  T4 : Trigonometry
  velocity_at_wheels_in_X_mux(4)final : Outport
  velocity_at_wheels_in_Y_mux(4)final : Outport  Port=2
  wires:
  T1/1 -> La7/2, La6/2
  Demux/2 -> La6/1
  T3/1 -> La4/2, La5/2
  Sum1/1 -> Mux1/2
  La6/1 -> Sum1/2
  La5/1 -> Sum1/1
  Sum3/1 -> Mux1/1
  La3/1 -> Sum3/2
  La2/1 -> Sum3/1
  Demux1/2 -> La7/1, La5/1
  Sum2/1 -> Mux6/2
  La7/1 -> Sum2/2
  La4/1 -> Sum2/1
  Sum4/1 -> Mux6/1
  La1/1 -> Sum4/2
  T4/1 -> La1/2, La3/2
  Demux1/1 -> La1/1, La2/1
  La/1 -> Sum4/1
  T2/1 -> La/2, La2/2
  Demux/1 -> La4/1, La3/1, La/1
  angel_of_rotation_of_front_Right_wheel/1 -> T1/1, T3/1
  angel_of_rotation_of_front_left_wheel/1 -> T4/1, T2/1
  Mux1/1 -> velocity_at_wheels_in_Y_mux(4)final/1
  Mux6/1 -> velocity_at_wheels_in_X_mux(4)final/1
  Demux1/4 -> Mux1/4
  Demux1/3 -> Mux1/3
  Demux/4 -> Mux6/4
  Demux/3 -> Mux6/3
  velocity_at_wheels_in_Y_mux(4)/1 -> Demux1/1
  velocity_at_wheels_in_X_mux(4)/1 -> Demux/1

== system Model_Platform/Vehicle model/Vehicle dynamics/velocity/velocity_at_Front_Left ==
  rate_of_change_Yaw_Angle : Inport
  longitudenal_velocity_Vx : Inport  Port=2
  Lateral_velocity_Vy : Inport  Port=3
  Divide : Product  Inputs=*/
  Length_CG_Front_Wheels : Constant  Value=Para.VD.Length_Front.v
  Product : Product  RndMeth=Zero
  Product1 : Product  RndMeth=Zero
  Rfl : Math  Operator=sqrt  SaturateOnIntegerOverflow=on
  Sum : Sum  Inputs=|++
  Sum1 : Sum  Inputs=|++
  Sum2 : Sum  Inputs=|++
  Sum3 : Sum  Inputs=|-+
  T1 : Trigonometry  Operator=cos
  T2 : Trigonometry
  ThetaFl : Trigonometry  Operator=atan
  Vfl/CG : Product  RndMeth=Zero
  Vfr/CGx : Product  RndMeth=Zero
  Vfr/CGy : Product  RndMeth=Zero
  Width_of_Car/2 : Constant  Value=Para.VD.Wheel_Base_Width.v/2
  pi : Constant  Value=pi
  velocity_at_Front_left_in_X : Outport
  velocity_at_Front_left_in_Y : Outport  Port=2
  wires:
  pi/1 -> Sum3/2
  Vfr/CGy/1 -> Sum2/1
  Vfr/CGx/1 -> Sum1/1
  Sum3/1 -> T1/1, T2/1
  T1/1 -> Vfr/CGx/2
  T2/1 -> Vfr/CGy/2
  Vfl/CG/1 -> Vfr/CGx/1, Vfr/CGy/1
  ThetaFl/1 -> Sum3/1
  Divide/1 -> ThetaFl/1
  Rfl/1 -> Vfl/CG/1
  Product1/1 -> Sum/2
  Width_of_Car/2/1 -> Product1/1, Product1/2, Divide/2
  Length_CG_Front_Wheels/1 -> Product/1, Product/2, Divide/1
  Product/1 -> Sum/1
  Sum/1 -> Rfl/1
  rate_of_change_Yaw_Angle/1 -> Vfl/CG/2
  Sum1/1 -> velocity_at_Front_left_in_X/1
  longitudenal_velocity_Vx/1 -> Sum1/2
  Sum2/1 -> velocity_at_Front_left_in_Y/1
  Lateral_velocity_Vy/1 -> Sum2/2

== system Model_Platform/Vehicle model/Vehicle dynamics/velocity/velocity_at_Front_Right ==
  rate_of_change_Yaw_Angle : Inport
  longitudenal_velocity_Vx : Inport  Port=2
  Lateral_velocity_Vy : Inport  Port=3
  Divide : Product  Inputs=*/
  Length_CG_Front_Wheels : Constant  Value=Para.VD.Length_Front.v
  Product : Product  RndMeth=Zero
  Product1 : Product  RndMeth=Zero
  Rfr : Math  Operator=sqrt  SaturateOnIntegerOverflow=on
  Sum : Sum  Inputs=|++
  Sum1 : Sum  Inputs=|++
  Sum2 : Sum  Inputs=|++
  ThetaFr : Trigonometry  Operator=atan
  ThetaFr1 : Trigonometry  Operator=cos
  ThetaFr2 : Trigonometry
  Vfr/CG : Product  RndMeth=Zero
  Vfr/CG1 : Product  RndMeth=Zero
  Vfr/CG2 : Product  RndMeth=Zero
  Width_of_Car/2 : Constant  Value=Para.VD.Wheel_Base_Width.v/2
  sign : Gain
  velocity_at_Front_Right_in_X : Outport
  velocity_at_Front_Right_in_Y : Outport  Port=2
  wires:
  Lateral_velocity_Vy/1 -> Sum2/2
  Sum2/1 -> velocity_at_Front_Right_in_Y/1
  longitudenal_velocity_Vx/1 -> Sum1/2
  Sum1/1 -> velocity_at_Front_Right_in_X/1
  rate_of_change_Yaw_Angle/1 -> Vfr/CG/2
  Sum/1 -> Rfr/1
  Product/1 -> Sum/1
  Length_CG_Front_Wheels/1 -> Divide/1, Product/2, Product/1
  Width_of_Car/2/1 -> Divide/2, Product1/2, Product1/1
  Product1/1 -> Sum/2
  Rfr/1 -> Vfr/CG/1
  Divide/1 -> ThetaFr/1
  ThetaFr/1 -> sign/1
  Vfr/CG/1 -> Vfr/CG2/1, Vfr/CG1/1
  ThetaFr2/1 -> Vfr/CG2/2
  ThetaFr1/1 -> Vfr/CG1/2
  sign/1 -> ThetaFr2/1, ThetaFr1/1
  Vfr/CG1/1 -> Sum1/1
  Vfr/CG2/1 -> Sum2/1

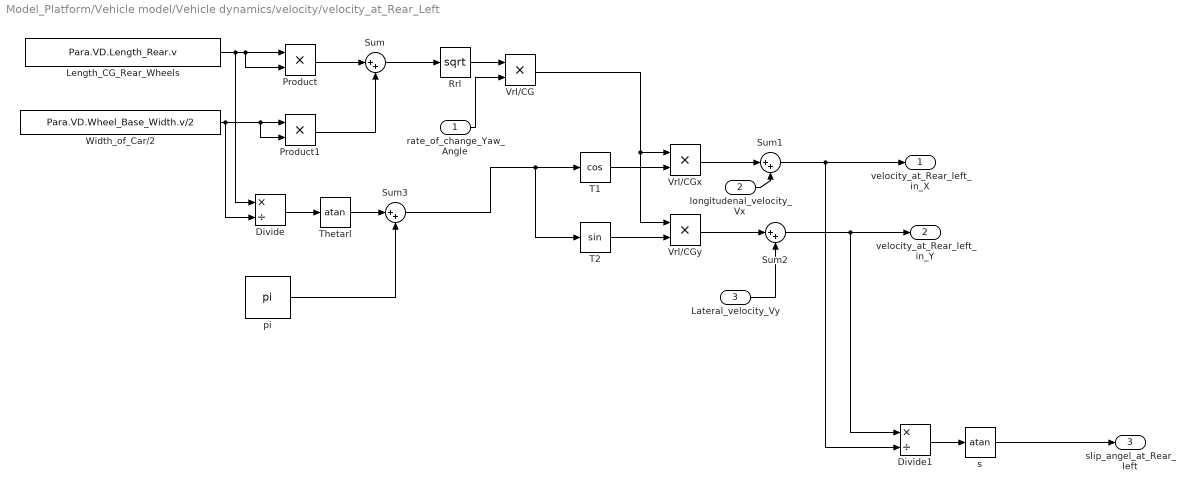
== system Model_Platform/Vehicle model/Vehicle dynamics/velocity/velocity_at_Rear_Left ==
  rate_of_change_Yaw_Angle : Inport
  longitudenal_velocity_Vx : Inport  Port=2
  Lateral_velocity_Vy : Inport  Port=3
  Divide : Product  Inputs=*/
  Divide1 : Product  Inputs=*/
  Length_CG_Rear_Wheels : Constant  Value=Para.VD.Length_Rear.v
  Product : Product  RndMeth=Zero
  Product1 : Product  RndMeth=Zero
  Rrl : Math  Operator=sqrt  SaturateOnIntegerOverflow=on
  Sum{,1..3} (4 alike) : Sum  Inputs=|++
  T1 : Trigonometry  Operator=cos
  T2 : Trigonometry
  Thetarl : Trigonometry  Operator=atan
  Vrl/CG : Product  RndMeth=Zero
  Vrl/CGx : Product  RndMeth=Zero
  Vrl/CGy : Product  RndMeth=Zero
  Width_of_Car/2 : Constant  Value=Para.VD.Wheel_Base_Width.v/2
  pi : Constant  Value=pi
  s : Trigonometry  Operator=atan
  velocity_at_Rear_left_in_X : Outport
  velocity_at_Rear_left_in_Y : Outport  Port=2
  slip_angel_at_Rear_left : Outport  Port=3
  wires:
  s/1 -> slip_angel_at_Rear_left/1
  Divide1/1 -> s/1
  pi/1 -> Sum3/2
  Lateral_velocity_Vy/1 -> Sum2/2
  Sum2/1 -> velocity_at_Rear_left_in_Y/1, Divide1/1
  longitudenal_velocity_Vx/1 -> Sum1/2
  Sum1/1 -> velocity_at_Rear_left_in_X/1, Divide1/2
  rate_of_change_Yaw_Angle/1 -> Vrl/CG/2
  Sum/1 -> Rrl/1
  Product/1 -> Sum/1
  Length_CG_Rear_Wheels/1 -> Divide/1, Product/2, Product/1
  Width_of_Car/2/1 -> Divide/2, Product1/2, Product1/1
  Product1/1 -> Sum/2
  Rrl/1 -> Vrl/CG/1
  Divide/1 -> Thetarl/1
  Thetarl/1 -> Sum3/1
  Vrl/CG/1 -> Vrl/CGy/1, Vrl/CGx/1
  T2/1 -> Vrl/CGy/2
  T1/1 -> Vrl/CGx/2
  Sum3/1 -> T2/1, T1/1
  Vrl/CGx/1 -> Sum1/1
  Vrl/CGy/1 -> Sum2/1

== system Model_Platform/Vehicle model/Vehicle dynamics/velocity/velocity_at_Rear_Right ==
  rate_of_change_Yaw_Angle : Inport
  longitudenal_velocity_Vx : Inport  Port=2
  Lateral_velocity_Vy : Inport  Port=3
  Divide : Product  Inputs=*/
  Length_CG_Rear_Wheels : Constant  Value=Para.VD.Length_Rear.v
  Product : Product  RndMeth=Zero
  Product1 : Product  RndMeth=Zero
  Rrr : Math  Operator=sqrt  SaturateOnIntegerOverflow=on
  Sum : Sum  Inputs=|++
  Sum1 : Sum  Inputs=|++
  Sum2 : Sum  Inputs=|++
  T1 : Trigonometry  Operator=cos
  T2 : Trigonometry
  Thetarr : Trigonometry  Operator=atan
  Vrr/CG : Product  RndMeth=Zero
  Vrr/CGx : Product  RndMeth=Zero
  Vrr/CGy : Product  RndMeth=Zero
  Width_of_Car/2 : Constant  Value=Para.VD.Wheel_Base_Width.v/2
  sign : Gain  Gain=-1
  velocity_at_Rear_Right_in_X : Outport
  velocity_at_Rear_Right_in_Y : Outport  Port=2
  wires:
  Vrr/CGy/1 -> Sum2/1
  Vrr/CGx/1 -> Sum1/1
  sign/1 -> T1/1, T2/1
  T1/1 -> Vrr/CGx/2
  T2/1 -> Vrr/CGy/2
  Vrr/CG/1 -> Vrr/CGx/1, Vrr/CGy/1
  Thetarr/1 -> sign/1
  Divide/1 -> Thetarr/1
  Rrr/1 -> Vrr/CG/1
  Product1/1 -> Sum/2
  Width_of_Car/2/1 -> Product1/1, Product1/2, Divide/2
  Length_CG_Rear_Wheels/1 -> Product/1, Product/2, Divide/1
  Product/1 -> Sum/1
  Sum/1 -> Rrr/1
  rate_of_change_Yaw_Angle/1 -> Vrr/CG/2
  Sum1/1 -> velocity_at_Rear_Right_in_X/1
  longitudenal_velocity_Vx/1 -> Sum1/2
  Sum2/1 -> velocity_at_Rear_Right_in_Y/1
  Lateral_velocity_Vy/1 -> Sum2/2

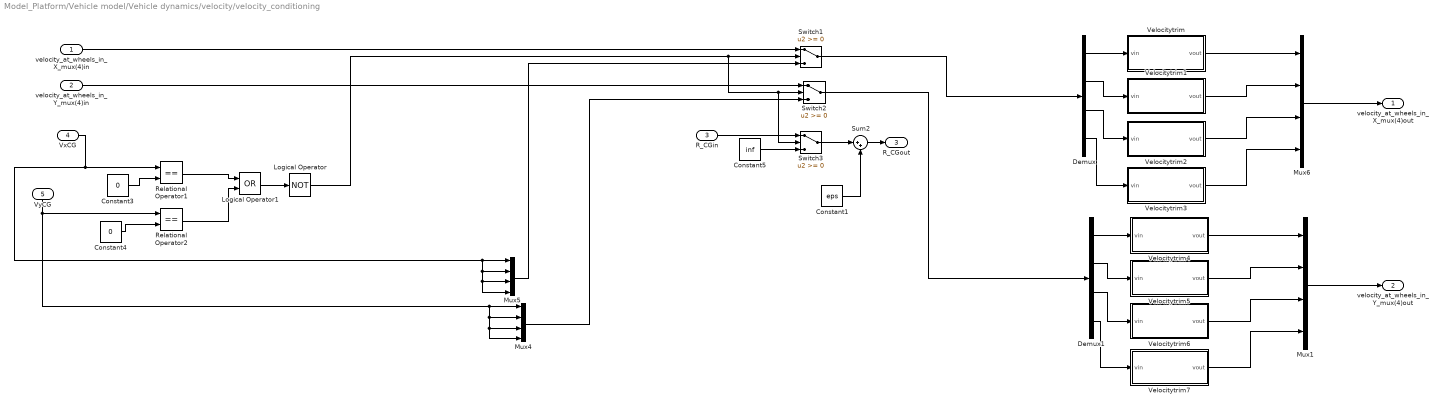
== system Model_Platform/Vehicle model/Vehicle dynamics/velocity/velocity_conditioning ==
  velocity_at_wheels_in_X_mux(4)in : Inport
  velocity_at_wheels_in_Y_mux(4)in : Inport  Port=2
  R_CGin : Inport  Port=3
  VxCG : Inport  Port=4
  VyCG : Inport  Port=5
  Constant1 : Constant  Value=eps
  Constant3 : Constant  Value=0
  Constant4 : Constant  Value=0
  Constant5 : Constant  Value=inf
  Demux : Demux
  Demux1 : Demux
  Logical Operator : Logic  Operator=NOT  AllPortsSameDT=off  OutDataTypeStr=boolean
  Logical Operator1 : Logic  Operator=OR  AllPortsSameDT=off  OutDataTypeStr=boolean
  Mux{1,4..6} (4 alike) : Mux
  Relational Operator1 : RelationalOperator  Operator===  OutDataTypeStr=boolean  RndMeth=Nearest
  Relational Operator2 : RelationalOperator  Operator===  OutDataTypeStr=boolean  RndMeth=Nearest
  Sum2 : Sum  Inputs=|++
  Switch1 : Switch
  Switch2 : Switch
  Switch3 : Switch
  Velocitytrim : Subsystem
  Velocitytrim1 : Subsystem
  Velocitytrim2 : Subsystem
  Velocitytrim3 : Subsystem
  Velocitytrim4 : Subsystem
  Velocitytrim5 : Subsystem
  Velocitytrim6 : Subsystem
  Velocitytrim7 : Subsystem
  velocity_at_wheels_in_X_mux(4)out : Outport
  velocity_at_wheels_in_Y_mux(4)out : Outport  Port=2
  R_CGout : Outport  Port=3
  wires:
  Switch2/1 -> Demux1/1
  Mux1/1 -> velocity_at_wheels_in_Y_mux(4)out/1
  Velocitytrim7/1(vout) -> Mux1/4
  Velocitytrim6/1(vout) -> Mux1/3
  Velocitytrim5/1(vout) -> Mux1/2
  Velocitytrim4/1(vout) -> Mux1/1
  Demux1/4 -> Velocitytrim7/1(vin)
  Demux1/3 -> Velocitytrim6/1(vin)
  Demux1/2 -> Velocitytrim5/1(vin)
  Demux1/1 -> Velocitytrim4/1(vin)
  Mux6/1 -> velocity_at_wheels_in_X_mux(4)out/1
  Switch1/1 -> Demux/1
  Velocitytrim3/1(vout) -> Mux6/4
  Velocitytrim2/1(vout) -> Mux6/3
  Velocitytrim1/1(vout) -> Mux6/2
  Velocitytrim/1(vout) -> Mux6/1
  Demux/4 -> Velocitytrim3/1(vin)
  Demux/3 -> Velocitytrim2/1(vin)
  Demux/2 -> Velocitytrim1/1(vin)
  Demux/1 -> Velocitytrim/1(vin)
  Sum2/1 -> R_CGout/1
  R_CGin/1 -> Switch3/1
  velocity_at_wheels_in_Y_mux(4)in/1 -> Switch2/1
  velocity_at_wheels_in_X_mux(4)in/1 -> Switch1/1
  VyCG/1 -> Mux4/4, Mux4/3, Mux4/2, Mux4/1, Relational Operator2/1
  VxCG/1 -> Relational Operator1/1, Mux5/4, Mux5/3, Mux5/2, Mux5/1
  Constant1/1 -> Sum2/2
  Switch3/1 -> Sum2/1
  Logical Operator1/1 -> Logical Operator/1
  Logical Operator/1 -> Switch3/2, Switch2/2, Switch1/2
  Constant5/1 -> Switch3/3
  Mux4/1 -> Switch2/3
  Mux5/1 -> Switch1/3
  Relational Operator2/1 -> Logical Operator1/2
  Relational Operator1/1 -> Logical Operator1/1
  Constant4/1 -> Relational Operator2/2
  Constant3/1 -> Relational Operator1/2
